simulink library "powerlib2"  (Simulink 6.0)
settings: Solver=ode45  SolverMode=SingleTasking  StartTime=0.0  StopTime=10.0  RelTol=1e-3
undefined symbols (not defined in the file or in its folder): com, ctrl1, Da, DiscIntNeverNeededParam, dtha, etat, FA, gcbh, Ha, Ka, Lm, Ls, powericonV2, q0, Rm, Rs, sel, st_a, st_b, st_c, sta, stb, stc, T1, T2, T3, T4
libraries: powerlib2 x55, simulink_extras x5, powerlib_extras x4, powerlib_modelsV2 x4, simulink x1
(part 1 of 6)
settings Model: Creator=patrice  LastModifiedBy=batserve  ExtModeAutoUpdateStatusClock=off
settings OptimizationCC: BooleanDataType=off
settings DebuggingCC: CheckExecutionContextPreStartOutputMsg=on  CheckExecutionContextRuntimeOutputMsg=on  SolverPrmCheckMsg=none
settings HardwareCC: TargetUnknown=on

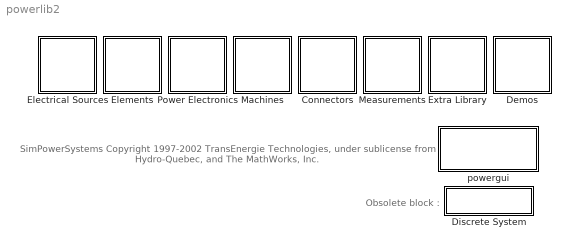
== system powerlib2 ==
  note: SimPowerSystems
      | Copyright  1997-2002 TransEnergie Technologies, under sublicense
      | from Hydro-Quebec, and The MathWorks, Inc.
  note: Obsolete block :
  Connectors : Subsystem
      mask Display: plot(0,0,100,100,[80,40],[40,40],[70,51],[31,31],[64,57],[23,23],[5,60,60],[70,70,40],[32,32],[70,97],[31,32,34,29,29,34,34,29,34,29],[71,68,71,71,70,68,71,68,68,71])
  Demos : Subsystem
      settings: OpenFcn=demo('simulink','SimPowerSystems')
      mask Display: disp('Demos')
  Discrete System : Subsystem  mask(PSB option block system){methode=0, Ts=50e-6}
      mask prompts: methode "methode (dummy)"; Ts "Sample time (s):"
      mask help:
      | This block is used to discretize the state-space model of a SimPowerSystems circuit, with the bilinear (Tustin) approximation.  Discrete time models will be used for Machine blocks and Power Electronics blocks.
      |
      | Drag this block in the top-level system of your model and specify the sample time.
      mask init:
      | if isempty(Ts);Ts=0;end;
      | if Ts==0
      |   message=sprintf('Continuous\nsystem');
      | else
      |   message=sprintf('Discrete system\nTs=%s',num2str(Ts));
      | end
      mask Help: web(psbhelp);
      mask Display: disp(message)
  Electrical Sources : Subsystem
      mask Display: plot(-15,-15,15,15,[0 0 5 -5],[10 1.25 1.25 1.25],[0 0 -2 2],[-10 -1.25 -1.25 -1.25],[6 4 5 5 5]-10,[3 3 3 4 2]+3)
  Elements : Subsystem  InitFcn=powericonV2('psblfblk',bdroot,'goto','Load');
      mask Display: plot(0,0,100,100,[90,64,77,77,60,56,51,46,40,34,30,25,13],[57,57,57,80,80,65,94,65,94,65,94,80,80],[90,87,82,77,74,68,64],[43,46,48,48,48,46,43],[48,77,77],[20,20,48],[39,27,13],[36,20,20])
  Extra Library : Subsystem
      settings: OpenFcn=powerlib_extras
      mask Display: disp('Extras')
  Machines : Subsystem
      mask Display: plot(-40,-40,40,40,[0,9,18,24,29,30,29,24,18,9,0,-9,-18,-24,-29,-30,-29,-24,-18,-9,0],[30,29,24,18,9,0,-9,-18,-24,-29,-30,-29,-24,-18,-9,0,9,18,24,29,30],[0,-9,-18,-24,-16,-16,-24,-18,-9,0,9,18,24,16,16,24,18,9,0]*.8,[-30,-29,-24,-18,-18,18,18,24,29,30,29,24,18,18,-18,-18,-24,-29,-30]*.8)
  Measurements : Subsystem  InitFcn=tag=strrep(tempname,tempdir,'');set_param(gcb,'VariableName',tag);
      mask Display: plot(-40,-40,40,60,[-30,-29,-24,-18,-9,0,9,18,24,29,30,-30],[0,9,18,24,29,30,29,24,18,9,0,0]*1.3,[0,10,3,10,12],[0,30,25,30,22])
  Power Electronics : Subsystem
      mask Display: plot(0,0,100,100,[50,30,70,50,30,70,50,50],[60,30,30,60,60,60,60,80],[50,50],[20,30],[30,41,44],[71,71,60])
  powergui : Subsystem  Priority=2  mask(PSB option menu block){Frange=[0:2:500], Ylog=off, Xlog=on, save=off, variable=ZData, structure=, ZoomFFT=on, StartTime=0.0, cycles=1, DisplayStyle=1, fundamental=60, FreqAxis=off, MaxFrequency=1000, frequencyindice=1, frequencyindicesteady=1, RmsSteady=1, display=off, Ts=0, methode=off, frequency=60, echomessages=off}
      mask prompts: Frange "Frequency Range (PSBZMETER)"; Ylog "Log impedance (PSBZMETER)"; Xlog "log Frequency (PSBZMETER)"; save "Save Data To Workspace (PSBZMETER)"; variable "Variable Name (PSBZMETER)"; structure "Structure Name (PSBFFTSCOPE)"; ZoomFFT "ZoomFFT (PSBFFTSCOPE)"; StartTime "Start Time (PSBFFTSCOPE)"; cycles "Cycles (PSBFFTSCOPE)"; DisplayStyle "Display style (PSBFFTSCOPE)"; fundamental "Fundamental (PSBFFTSCOPE)"; FreqAxis "Frequency Axis (PSBFFTSCOPE)"; MaxFrequency "Max Frequency (PSBFFTSCOPE)"; frequencyindice "Frequency indice  (PSBLOADFLOW)"; frequencyindicesteady "Frequency indice (STEADYSTATE)"; RmsSteady "RMS display (STEADYSTATE)"; display "Display Results"; Ts "Sample time (s):"; methode "Phasor simulation"; frequency "phasor frequency"; echomessages "Echo initialisation messages"
      mask init:
      | if isempty(Ts);Ts=-1;end;
      | if Ts==0
      |   message=sprintf('Powergui\n-Continuous');
      | elseif Ts>0
      |   message=sprintf('Powergui\n-Discrete,\nTs = %.4g s.',Ts);
      | else
      |   message=sprintf('Powergui\n-Discrete,\n Ts = ?');
      | end
      | if methode
      |     message=sprintf('Powergui\n-Phasors');
      | end
      | if strcmp(bdroot,'powerlib2')
      |   message='powergui';
      | end
      | if strcmp(bdroot,'powerlib')
      |   message='powergui';
      | end
      settings: DeleteFcn=close(get_param(gcbh,'userdata'))  OpenFcn=powergui(gcb)  CloseFcn=close(get_param(gcbh,'userdata'))
      mask Display: disp(message)

== system powerlib2/Connectors ==
  Bus Bar (horiz) : Subsystem  Tag=PoWeRsYsTeMbLoCk  Orientation=down  mask(Bus Bar){entrees=2, sorties=1, PSBOutputType=1111111111111111111111111111111111111111111111111111111111111111111111111}
      mask prompts: entrees "Number of inputs:"; sorties "Number of outputs:"; PSBOutputType "Output type [1=PSB  0=simulink output]"
      mask help: Use this block to connect multiple incoming lines together.
      mask init:
      | ret=powericonV2('Bus Bar',entrees,sorties);
      mask Help: web(psbhelp);
      mask Display: plot(0,0,10,ret)
  Bus Bar (thin horiz) : Subsystem  Tag=PoWeRsYsTeMbLoCk  Orientation=down  mask(Bus Bar){input=2, output=1, PSBOutputType=111111111111111111111111111111111111111111111111111111111111111111111111111111111111}
      mask prompts: input "Number of inputs:"; output "Number of outputs:"; PSBOutputType "Output type [1=PSB  0=simulink output]"
      mask help: Use this block to connect multiple incoming lines together.
      mask init:
      | [s,c1,c2] = powericonV2('Bus Bar',input,output);
      settings: CopyFcn=set_param(gcbh,'ShowName','off');
      mask Help: web(psbhelp);
      mask Display: plot(0,0,10,s,c1,c2)
  Bus Bar (thin vert) : Subsystem  Tag=PoWeRsYsTeMbLoCk  mask(Bus Bar){input=2, output=2, PSBOutputType=111111111111111111111111111111111111111111111111111111111111111111111111111111111111}
      mask prompts: input "Number of inputs:"; output "Number of outputs:"; PSBOutputType "Output type [1=PSB  0=simulink output]"
      mask help: Use this block to connect multiple incoming lines together.
      mask init:
      | [s,c1,c2] = powericonV2('Bus Bar',input,output);
      settings: CopyFcn=set_param(gcbh,'ShowName','off');
      mask Help: web(psbhelp);
      mask Display: plot(0,0,10,s,c1,c2)
  Bus Bar (vert) : Subsystem  Tag=PoWeRsYsTeMbLoCk  mask(Bus Bar){entrees=3, sorties=2, PSBOutputType=11111111111111111111111111111111111111111111111111111111111111111111111111111111111111111}
      mask prompts: entrees "Number of inputs:"; sorties "Number of outputs:"; PSBOutputType "Output type [1=PSB  0=simulink output]"
      mask help: Use this block to connect multiple incoming lines together.
      mask init:
      | ret=powericonV2('Bus Bar',entrees,sorties);
      mask Help: web(psbhelp);
      mask Display: plot(0,0,10,ret)
  Ground (input) : Subsystem  Tag=PoWeRsYsTeMbLoCk  Orientation=down
      settings: CopyFcn=set_param(gcbh,'ShowName','off');
      mask Type: Ground
      mask Description: Ground connection.
      mask Help: web(psbhelp);
      mask Display: plot(-15,-15,15,15,-[5 5],[-10 10],[0 0],[-5 5],-[-5 -5],[-2.5 2.5],-[15 5],[0 0])
  Ground (output) : Subsystem  Tag=PoWeRsYsTeMbLoCk  Orientation=up  mask(Ground){PSBOutputType=1}
      mask prompts: PSBOutputType "Output type [1=PSB  0=simulink output]"
      mask help: Ground connection
      settings: CopyFcn=set_param(gcbh,'ShowName','off');
      mask Help: web(psbhelp);
      mask Display: plot(-15,-15,15,15,[5 5],[-10 10],[0 0],[-5 5],[-5 -5],[-2.5 2.5],[15 5],[0 0])
  L connector : Subsystem  Tag=PoWeRsYsTeMbLoCk  TreatAsAtomicUnit=on  mask(Bus Bar){}
      mask help: Use this block to connect two incoming lines together.
      mask init:
      | if strcmp(get_param(gcb,'NamePlacement'),'alternate')
      |    rot = -1;
      | else
      |    rot = 1;
      | end
      settings: CopyFcn=set_param(gcbh,'ShowName','off');
      mask Help: web(psbhelp);
      mask Display:
      | plot(-100,-100,100,100,[-100,0,0],rot*[0,0,100])
      | plot([0 1 0 0 1 1 0 1]*30-10,[1 1 0 1 0 1 0 0]*30-15)
  Neutral (input) : Subsystem  Tag=PoWeRsYsTeMbLoCk  Orientation=down  mask(Neutral){no=99}
      mask prompts: no "Node number:"
      mask help: Implements a neutral point with a labeled number
      mask init:
      | strno=sprintf('\n\n%d',no);
      settings: CopyFcn=set_param(gcbh,'ShowName','off');
      mask Help: web(psbhelp);
      mask Display:
      | plot(-10,-10,10,10,-[10 5 5 -5 5 5],[0 0 -5 0 5 0.0])
      | disp(strno);
  Neutral (output) : Subsystem  Tag=PoWeRsYsTeMbLoCk  Orientation=up  mask(Neutral){no=99, PSBOutputType=1}
      mask prompts: no "Node number:"; PSBOutputType "Output type [1=PSB  0=simulink output]"
      mask help: Implements a neutral point with a labeled number
      mask init:
      | strno=sprintf('\n\n%d',no);
      settings: CopyFcn=set_param(gcbh,'ShowName','off');
      mask Help: web(psbhelp);
      mask Display:
      | plot(-10,-10,10,10,[10 5 5 -5 5 5],[0 0 -5 0 5 0.0])
      | disp(strno);
  T connector : Subsystem  Tag=PoWeRsYsTeMbLoCk  TreatAsAtomicUnit=on  mask(Bus Bar){PSBOutputType=1}
      mask prompts: PSBOutputType "Output type [1=PSB  0=simulink output]"
      mask help: Use this block to connect two incoming lines together.
      mask init:
      | if strcmp(get_param(gcb,'NamePlacement'),'alternate')
      |    rot = -1;
      | else
      |    rot = 1;
      | end
      settings: CopyFcn=set_param(gcbh,'ShowName','off');
      mask Help: web(psbhelp);
      mask Display:
      | plot(-100,-100,100,100,[-100 100],[0 0])
      | plot([0 0],rot*[100 0])
      | plot([0 1 0 0 1 1 0 1]*30-10,[1 1 0 1 0 1 0 0]*30-15)

== system powerlib2/Demos ==

== system powerlib2/Discrete System ==

== system powerlib2/Electrical Sources ==
  3-Phase  Programmable  Voltage Source : Subsystem  InitFcn=powericonV2('psbcbtransfo',gcb,'3-PhaseProgrammableVoltageSource',1);  mask(3-phase Programmable Voltage Source){Par_Vps_LLrms=[25e3 -20  60], VariationEntity=None, VariationType=Modulation, VariationStep=-0.3, VariationRate=0.5, VariationMag=0.4, VariationFreq=2, Par_Timing_Variation=[0.1 1.2], SinglePhase=off, Yampli=[1  0.8  1.2  1.0 ], Xtime=[0 0.1 0.25 0.4], HarmonicGeneration=off, Par_HarmoA_pu=[3 0.2 -25 0], Par_HarmoB_pu=[2 0.15  35 2], Par_Timing_Harmo=[0.1  0.6]}
      mask prompts: Par_Vps_LLrms "Positive-sequence: [ Amplitude(Vrms Ph-Ph)  Phase(deg.)   Freq. (Hz) ]"; VariationEntity "Time variation of:"; VariationType "Type of variation:"; VariationStep "Step magnitude (pu, Hz or deg.):"; VariationRate "Rate of change (pu/s, Hz/s or deg/s):"; VariationMag "Amplitude of the modulation (pu, Hz or deg.):"; VariationFreq "Frequency of the modulation(Hz):"; Par_Timing_Variation "Variation timing (s) : [ Start   End ]"; SinglePhase "Variation on phase A only"; Yampli "Amplitude values (pu):"; Xtime "Time values:"; HarmonicGeneration "Fundamental and/or Harmonic generation:"; Par_HarmoA_pu "A:  [ Order(n)   Amplitude(pu)  Phase(deg.)  Seq(0, 1 or 2) ]"; Par_HarmoB_pu "B:  [ Order(n)   Amplitude(pu)  Phase(deg.)  Seq(0, 1 or 2) ]"; Par_Timing_Harmo "Timing (s) : [ Start   End ]"
      mask help:
      | This block implements  a  three-phase zero-impedance voltage source. The common node (neutral) of the three sources is accessible via input 1 (N) of the block. Time variation for the amplitude, phase and frequency of the fundamental can be pre-programmed. In addition, two harmonics can be surimposed on the fundamental.
      |
      | Note: For  "Phasor simulation" , frequency variation and harmonic injection are not allowed.  Specify  Order =1 and Seq=1,2 or 0 to inject additional fundamendal components A and B in  any sequence.
      mask init:
      | % Conversion of pos. seq.amplitude from Ph-Ph rms voltage to Ph-G peak
      | Par_Vps=Par_Vps_LLrms;
      | Par_Vps(1)=Par_Vps(1)*sqrt(2/3);
      | Mag_Vps=Par_Vps(1);
      | Phase_Vps=Par_Vps(2);
      | Freq_Vps=Par_Vps(3);
      | % Conversion of harmonic amplitudes from pu to Ph-G peak volt
      | Par_HarmoA=Par_HarmoA_pu;
      | Par_HarmoB=Par_HarmoB_pu;
      | Par_HarmoA(2)=Par_HarmoA(2)*Mag_Vps;
      | Par_HarmoB(2)=Par_HarmoB(2)*Mag_Vps;
      | % Conversion of amplitude variation from pu to Ph-G peak volt
      | if VariationEntity==2
      | 	VariationStep=VariationStep*Mag_Vps;
      | 	VariationRate=VariationRate*Mag_Vps;
      | 	VariationMag=VariationMag*Mag_Vps;
      | 	Yampli=Yampli*Mag_Vps;
      | end
      | 
      | Ton_Variation=Par_Timing_Variation(1);
      | Toff_Variation=Par_Timing_Variation(2);
      | n_HarmoA=Par_HarmoA(1);
      | Mag_HarmoA=Par_HarmoA(2);
      | Phase_HarmoA=Par_HarmoA(3);
      | Seq_HarmoA=Par_HarmoA(4);
      | if n_HarmoA==0
      |     Phase_HarmoA=90;
      |     Seq_HarmoA=0;
      | end
      | n_HarmoB=Par_HarmoB(1);
      | Mag_HarmoB=Par_HarmoB(2);
      | Phase_HarmoB=Par_HarmoB(3);
      | Seq_HarmoB=Par_HarmoB(4);
      | if n_HarmoB==0
      |     Phase_HarmoB=90;
      |     Seq_HarmoB=0;
      | end
      | Ton_Harmo=Par_Timing_Harmo(1);
      | Toff_Harmo=Par_Timing_Harmo(2);
      | if length(Yampli) ~= length(Xtime),
      |    h=errordlg(' The vectors specifying the time and amplitude pairs must have the same length ' , 'Parameter error');
      | end
      | if Xtime(1)~=0,
      |    h=errordlg(' A pair time-amplitude must be specified at time zero' , 'Parameter error');
      | Xtime=[0 Xtime];
      | Yampli=[0 Yampli];
      | end
      | n=length(Xtime); vec_dt= [Xtime,0] - [0,Xtime] ; vec_dt=vec_dt(2:n);
      | if any(vec_dt<=0)
      |    h=errordlg(' All transition times must be in increasing order' , 'Parameter error');
      | end
      | if (VariationType==4 & VariationEntity>2),
      |      h=errordlg(' This type of variation (Table of time-amplitude pairs) is not valid for a variation of phase or frequency' , 'Parameter error');
      | end
      mask Help: web(psbhelp)
      mask StyleString: edit,popup(None|Amplitude|Phase|Frequency),popup(Step|Ramp|Modulation|Table of time-amplitude pairs),edit,edit,edit,edit,edit,checkbox,edit,edit,checkbox,edit,edit,edit
      mask CallbackString: |parametres=get_param(gcb,'MaskValues');p2=parametres{2};p3=parametres{3};p12=parametres{12};if strcmp(p3,'Step');param4='on';param5='off';param6='off';param7='off';param8='on';param9='off';param10='off';param11='off';elseif strcmp(p3,'Ramp');param4='off';param5='on';param6='off';param7='off';param8='on';param9='off';param10='off';param11='off';elseif strcmp(p3,'Modulation');param4='off';param5='off';param6='on';param7='on';param8='on';param9='off';param10='off';param11='off';else;param4='off';param5='off';param6='off';param7='off';param8='off';param9='on';param10='on';param11='on';end;if strcmp(p2,'None');param3='off';param4='off';param5='off';param6='off';param7='off';param8='off';param9='off';param10='off';param11='off';else;param3='on';end;if strcmp(p12,'on');param13='on';param14='on';param15='on';else;param13='off';param14='off';param15='off';end;visible={'on','on',param3,param4,param5,param6,param7,param8,param9,param10,param11,'on',param13,param14,param15};set_param(gcb,'MaskVisibilities',visible)|parametres=get_param(gcb,'MaskValues');p2=parametres{2};p3=parametres{3};p12=parametres{12};if strcmp(p3,'Step');param4='on';param5='off';param6='off';param7='off';param8='on';param9='off';param10='off';param11='off';elseif strcmp(p3,'Ramp');param4='off';param5='on';param6='off';param7='off';param8='on';param9='off';param10='off';param11='off';elseif strcmp(p3,'Modulation');param4='off';param5='off';param6='on';param7='on';param8='on';param9='off';param10='off';param11='off';else;param4='off';param5='off';param6='off';param7='off';param8='off';param9='on';param10='on';param11='on';end;if strcmp(p2,'None');param3='off';param4='off';param5='off';param6='off';param7='off';param8='off';param9='off';param10='off';param11='off';else;param3='on';end;if strcmp(p12,'on');param13='on';param14='on';param15='on';else;param13='off';param14='off';param15='off';end;visible={'on','on',param3,param4,param5,param6,param7,param8,param9,param10,param11,'on',param13,param14,param15};set_param(gcb,'MaskVisibilities',visible)|||||||||parametres=get_param(gcb,'MaskValues');p2=parametres{2};p3=parametres{3};p12=parametres{12};if strcmp(p3,'Step');param4='on';param5='off';param6='off';param7='off';param8='on';param9='off';param10='off';param11='off';elseif strcmp(p3,'Ramp');param4='off';param5='on';param6='off';param7='off';param8='on';param9='off';param10='off';param11='off';elseif strcmp(p3,'Modulation');param4='off';param5='off';param6='on';param7='on';param8='on';param9='off';param10='off';param11='off';else;param4='off';param5='off';param6='off';param7='off';param8='off';param9='on';param10='on';param11='on';end;if strcmp(p2,'None');param3='off';param4='off';param5='off';param6='off';param7='off';param8='off';param9='off';param10='off';param11='off';else;param3='on';end;if strcmp(p12,'on');param13='on';param14='on';param15='on';else;param13='off';param14='off';param15='off';end;visible={'on','on',param3,param4,param5,param6,param7,param8,param9,param10,param11,'on',param13,param14,param15};set_param(gcb,'MaskVisibilities',visible)|||
      mask Display:
      | plot(-50,-35,50,50-15,[0,9,18,24,29,30,29,24,18,9,0,-9,-18,-24,-29,-30,-29,-24,-18,-9,0],[30,29,24,18,9,0,-9,-18,-24,-29,-30,-29,-24,-18,-9,0,9,18,24,29,30],[-50 -30],[0 0],[50,30],[0 0],[45 35 40 40 40],[15 15 15 20 10],[1 2 3 4 5 6 7 8 9 10 11 12 13 14 15 16 17 18 19 20 21].*1.5-15,[0,9,18,24,29,30,29,24,18,9,0,-9,-18,-24,-29,-30,-29,-24,-18,-9,0]./2.4)
      | plot(-75,-70,75,70)
  3-Phase Source : Subsystem  Tag=PoWeRsYsTeMbLoCk  mask(3-Phase Source){V=25e3, Phi=0, F=60, InternalConnection=Yn, RLoff=on, R=0.312, L=6.63e-3, Psc=0, Vbase=0, XRratio=0, PSBOutputType=111}
      mask prompts: V "Phase-to-phase rms voltage (V):"; Phi "Phase angle of phase A (degrees):"; F "Frequency (Hz) :"; InternalConnection "Internal connection:"; RLoff "Specify impedance using short-circuit level"; R "Source resistance (Ohms):"; L "Source inductance (H) :"; Psc "3-phase short-circuit level at base voltage(VA):"; Vbase "Base voltage (Vrms ph-ph):"; XRratio "X/R ratio:"; PSBOutputType "Output type [1=PSB  0=simulink output]"
      mask help: This block implements a three-phase source in series with a serie RL branch.
      mask init:
      | parametres=get_param(gcb,'MaskValues');
      | p5=parametres{5};
      | if strcmp(p5,'on');
      |         param6='off';
      |         param7='off';
      |         param8='on';
      |         param9='on';
      |         param10='on';
      |         param11='off';
      | else 
      |         param6='on';
      |         param7='on';
      |         param8='off';
      |         param9='off';
      |         param10='off';
      |         param11='off';
      | end
      | visible={'on','on','on','on','on',param6,param7,param8,param9,param10,param11};
      | set_param(gcb,'MaskVisibilities',visible);
      |     %
      | WantYn = strcmp(get_param(gcb,'InternalConnection'),'Yn');
      | ports = get_param(gcb,'ports');
      | External = (ports(1)==1);
      |     %
      | if WantYn & ~External
      |         replace_block(gcb,'Followlinks','on','Name','N','Inport','noprompt');
      | elseif ~WantYn & External 
      |         replace_block(gcb,'Followlinks','on','Name','N','Constant','noprompt');
      | end
      | %
      | [s1,s2,s3,s4]=powericonV2('3-phase inductive source - Ungrounded neutral',R,L);
      | %
      | if InternalConnection==3
      | 	g1 = [-150,-150];
      | 	g2 = [-15,15];
      | 	g3 = [-165,-165];
      | 	g4 = [-10,10];
      | 	g5 = [-180,-180];
      | 	g6 = [-5,5];
      | else
      | 	g1=0;g2=0;g3=0;g4=0;g5=0;g6=0;
      | end
      mask Help: Three-phase voltage source with source resistance and inductance.
      mask StyleString: edit,edit,edit,popup(Y|Yn|Yg),checkbox,edit,edit,edit,edit,edit,edit
      mask CallbackString:
      | |||parametres=get_param(gcb,'MaskValues');
      | p5=parametres{5};
      | if strcmp(p5,'on');
      |         param6='off';
      |         param7='off';
      |         param8='on';
      |         param9='on';
      |         param10='on';
      |         param11='off';
      | else
      |         param6='on';
      |         param7='on';
      |         param8='off';
      |         param9='off';
      |         param10='off';
      |         param11='off';
      | end
      | visible={'on','on','on','on','on',param6,param7,param8,param9,param10,param11};
      | set_param(gcb,'MaskVisibilities',visible);
      |     %
      | WantYn = strcmp(get_param(gcb,'InternalConnection'),'Yn');
      | ports = get_param(gcb,'ports');
      | External = (ports(1)==1);
      |     %
      | if WantYn & ~External
      |         replace_block(gcb,'Followlinks','on','Name','N','Inport','noprompt');
      | elseif ~WantYn & External
      |         replace_block(gcb,'Followlinks','on','Name','N','Constant','noprompt');
      | end |parametres=get_param(gcb,'MaskValues');
      | p5=parametres{5};
      | if strcmp(p5,'on');
      |         param6='off';
      |         param7='off';
      |         param8='on';
      |         param9='on';
      |         param10='on';
      |         param11='off';
      | else
      |         param6='on';
      |         param7='on';
      |         param8='off';
      |         param9='off';
      |         param10='off';
      |         param11='off';
      | end
      | visible={'on','on','on','on','on',param6,param7,param8,param9,param10,param11};
      | set_param(gcb,'MaskVisibilities',visible);
      |     %
      | WantYn = strcmp(get_param(gcb,'InternalConnection'),'Yn');
      | ports = get_param(gcb,'ports');
      | External = (ports(1)==1);
      |     %
      | if WantYn & ~External
      |         replace_block(gcb,'Followlinks','on','Name','N','Inport','noprompt');
      | elseif ~WantYn & External
      |         replace_block(gcb,'Followlinks','on','Name','N','Constant','noprompt');
      | end||||||
      mask Display:
      | plot(-180,-50,360,50,s1,s2,s3,s4,
      | [0,9,18,24,29,30,29,24,18,9,0,-9,-18,-24,-29,-30,-29,-24,-18,-9,0]*1.5-45,
      | [30,29,24,18,9,0,-9,-18,-24,-29,-30,-29,-24,-18,-9,0,9,18,24,29,30]*0.8,[-150,-90],[0,0]);
      | plot(g1,g2,g3,g4,g5,g6);
  AC Current Source : Subsystem  Tag=PoWeRsYsTeMbLoCk  Description=source block  Orientation=up  LoadFcn=powericonV2('psblfblk',bdroot,'goto','Load');  mask(AC Current Source){A=10, P=0, F=60, stime=0, mesure=None, PSBOutputType=1}
      mask prompts: A "Peak amplitude (A):"; P "Phase (deg):"; F "Frequency (Hz):"; stime "Sample time:"; mesure "Measurements"; PSBOutputType "Output type [1=PSB  0=simulink output]"
      mask help: Ideal sinusoidal AC current source. The positive current direction is indicated by the arrow.
      settings: CopyFcn=powericonV2('psblfblk',bdroot,'goto','Copy');
      mask Help: web(psbhelp);
      mask StyleString: edit,edit,edit,edit,popup(None|Current),edit
      mask Display: plot(-50,-35,50,50-15,[0,9,18,24,29,30,29,24,18,9,0,-9,-18,-24,-29,-30,-29,-24,-18,-9,0],[30,29,24,18,9,0,-9,-18,-24,-29,-30,-29,-24,-18,-9,0,9,18,24,29,30],[-20 5 5 20 5 5],[2 2 12 2 -8 2],[-50 -30],[0 0],[50,30],[0 0],[45 35 40 40 40],[15 15 15 20 10]);
  AC Voltage Source : Subsystem  Tag=PoWeRsYsTeMbLoCk  Description=source block  Orientation=up  LoadFcn=powericonV2('psblfblk',bdroot,'goto','Load');  mask(AC Voltage Source){A=100, P=0, F=60, stime=0, mesure=None, PSBOutputType=1}
      mask prompts: A "Peak amplitude (V):"; P "Phase (deg):"; F "Frequency (Hz):"; stime "Sample time:"; mesure "Measurements"; PSBOutputType "Output type [1=PSB  0=simulink output]"
      mask help: Ideal sinusoidal AC Voltage source.
      settings: CopyFcn=powericonV2('psblfblk',bdroot,'goto','Copy');
      mask Help: web(psbhelp);
      mask StyleString: edit,edit,edit,edit,popup(None|Voltage),edit
      mask Display: plot(-50,-35,50,50-15,[0,9,18,24,29,30,29,24,18,9,0,-9,-18,-24,-29,-30,-29,-24,-18,-9,0],[30,29,24,18,9,0,-9,-18,-24,-29,-30,-29,-24,-18,-9,0,9,18,24,29,30],[-50 -30],[0 0],[50,30],[0 0],[45 35 40 40 40],[15 15 15 20 10],[0,9,18,24,29,30,29,24,18,9,0,-9,-18,-24,-29,-30,-29,-24,-18,-9,0]./-2.4,[1 2 3 4 5 6 7 8 9 10 11 12 13 14 15 16 17 18 19 20 21].*1.5-15);
  Controlled Current Source : Subsystem  Tag=PoWeRsYsTeMbLoCk  Description=source block  LoadFcn=powericonV2('psblfblk',bdroot,'goto','Load');  mask(Controlled Current Source){initsrc=on, srctyp=AC, ia=0, iph=0, freq=0, mesure=None, PSBOutputType=11}
      mask prompts: initsrc "Initialize"; srctyp "Source type"; ia "Initial amplitude (A):"; iph "Initial phase (deg):"; freq "Initial frequency (Hz):"; mesure "Measurements"; PSBOutputType "Output type [1=PSB  0=simulink output]"
      mask help:
      | Converts the Simulink input signal into an equivalent current source. The generated current is driven by the input signal of the block.
      |
      | You can initialize your circuit with a specific AC or DC current. If you want to start the simulation in steady-state, the block input must be connected to a signal starting as a sinusoidal or DC waveform corresponding to the initial values.
      mask init:
      | powericonV2('psbcbtransfo',gcb,'CCS:initialize');
      settings: CopyFcn=powericonV2('psblfblk',bdroot,'goto','Copy');
      mask Help: web(psbhelp);
      mask StyleString: checkbox,popup(AC|DC),edit,edit,edit,popup(None|Current),edit
      mask CallbackString: powericonV2('psbcbtransfo',gcb,'CCS:initialize');|powericonV2('psbcbtransfo',gcb,'CCS:source type');|||||
      mask Display:
      | plot(0,0,100,100)
      | plot([50 50 40  50 60 50]+35,[ 30,70,70,80,70,70]);
  Controlled Voltage Source : Subsystem  Tag=PoWeRsYsTeMbLoCk  Description=source block  LoadFcn=powericonV2('psblfblk',bdroot,'goto','Load');  mask(Controlled Voltage Source){initsrc=on, srctyp=AC, iv=0, iph=0, ifreq=0, mesure=None, PSBOutputType=11}
      mask prompts: initsrc "Initialize"; srctyp "Source type"; iv "Initial amplitude (V):"; iph "Initial phase (deg):"; ifreq "Initial frequency (Hz):"; mesure "Measurements"; PSBOutputType "Output type [1=PSB  0=simulink output]"
      mask help:
      | Converts the Simulink input signal into an equivalent voltage source. The generated voltage is driven by the input signal of the block.
      |
      | You can initialize your circuit with a specific AC or DC voltage. If you want to start the simulation in steady-state, the block input must be connected to a signal starting as a sinusoidal or DC waveform corresponding to the initial values.
      mask init:
      | powericonV2('psbcbtransfo',gcb,'CCS:initialize');
      settings: CopyFcn=powericonV2('psblfblk',bdroot,'goto','Copy');
      mask Help: web(psbhelp);
      mask StyleString: checkbox,popup(AC|DC),edit,edit,edit,popup(None|Voltage),edit
      mask CallbackString: powericonV2('psbcbtransfo',gcb,'CCS:initialize');|powericonV2('psbcbtransfo',gcb,'CCS:source type');|||||
  DC Voltage Source : Subsystem  Tag=PoWeRsYsTeMbLoCk  Description=source block  Orientation=up  LoadFcn=powericonV2('psblfblk',bdroot,'goto','Load');  mask(DC Voltage Source){V=100, mesure=None, PSBOutputType=1}
      mask prompts: V "Amplitude (V):"; mesure "Measurements"; PSBOutputType "Output type [1=PSB  0=simulink output]"
      mask help: Ideal DC voltage source.
      settings: CopyFcn=powericonV2('psblfblk',bdroot,'goto','Copy');
      mask Help: web(psbhelp);
      mask StyleString: edit,popup(None|Voltage),edit
      mask Display: plot(-10,-5,10,5,[10 1.25 1.25 1.25],[0 0 5 -5],[-10 -1.25 -1.25 -1.25],[0 0 -2 2],[6 4 5 5 5],[3 3 3 4 2])
